simulink model "manipulator2"  (Simulink 8.8)
settings: Solver=FixedStepAuto  StartTime=0.0  StopTime=10.2557  FixedStep=0.001  RelTol=1e-3
settings Model: Creator=dell  LastModifiedBy=dell
settings DataIOCC: LimitDataPoints=off  SaveFormat=Dataset  SignalLoggingSaveFormat=Dataset
settings OptimizationCC: LifeSpan=auto
settings DebuggingCC: UnderspecifiedInitializationDetection=Simplified  MergeDetectMultiDrivingBlocksExec=error  FcnCallInpInsideContextMsg=error  StateNameClashWarn=none  SFUnexpectedBacktrackingDiag=error  SFNoUnconditionalDefaultTransitionDiag=error  SFExecutionAtInitializationDiag=warning
settings HardwareCC: ProdBitPerPointer=64  ProdBitPerSizeT=64  ProdBitPerPtrDiffT=64  ProdLargestAtomicFloat=Float  ProdIntDivRoundTo=Zero  ProdEndianess=LittleEndian  ProdWordSize=64  ProdHWDeviceType=Intel->x86-64 (Windows64)
settings ModelReferenceCC: PropagateSignalLabelsOutOfModel=on
settings GRTTargetCC: TargetLangStandard=C99 (ISO)  GeneratePreprocessorConditionals=Use local settings  CombineOutputUpdateFcns=on  GRTInterface=off
settings ConfigComp: CovMetricSettings=dwe  CovHtmlReporting=off  CovSaveCumulativeToWorkspaceVar=off  CovSaveSingleToWorkspaceVar=off  CovExternalEMLEnable=on

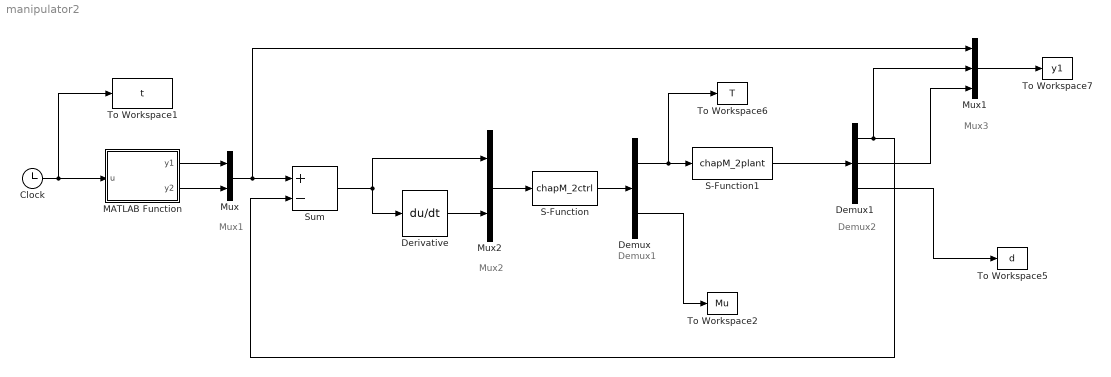
== system manipulator2 ==
  note: Demux2
  note: Mux3
  note: Demux1
  note: Mux2
  note: Mux1
  Clock : Clock
  Demux : Demux  Outputs=2
  Demux1 : Demux  Outputs=3
  Derivative : Derivative
  MATLAB Function : MATLAB Function  TreatAsAtomicUnit=on
  Mux : Mux  Inputs=2
  Mux1 : Mux  Inputs=3
  Mux2 : Mux  Inputs=2
  S-Function : S-Function  FunctionName=chapM_2ctrl  SFunctionDeploymentMode=off  EnableBusSupport=off
  S-Function1 : S-Function  FunctionName=chapM_2plant  SFunctionDeploymentMode=off  EnableBusSupport=off
  Sum : Sum  Inputs=+-  SaturateOnIntegerOverflow=on  InputSameDT=on  OutDataTypeStr=Inherit: Same as first input
  To Workspace1 : ToWorkspace  VariableName=t  SampleTime=-1
  To Workspace2 : ToWorkspace  VariableName=Mu  SampleTime=-1
  To Workspace5 : ToWorkspace  VariableName=d  SampleTime=-1
  To Workspace6 : ToWorkspace  VariableName=T  SampleTime=-1
  To Workspace7 : ToWorkspace  VariableName=y1  SampleTime=-1
  wires:
  MATLAB Function/2(y2) -> Mux/2
  MATLAB Function/1(y1) -> Mux/1
  S-Function/1 -> Demux/1
  Demux/1 -> To Workspace6/1, S-Function1/1
  S-Function1/1 -> Demux1/1
  Clock/1 -> To Workspace1/1, MATLAB Function/1(u)
  Mux2/1 -> S-Function/1
  Derivative/1 -> Mux2/2
  Mux1/1 -> To Workspace7/1
  Mux/1 -> Mux1/1, Sum/1
  Sum/1 -> Mux2/1, Derivative/1
  Demux/2 -> To Workspace2/1
  Demux1/3 -> To Workspace5/1
  Demux1/1 -> Mux1/2, Sum/2
  Demux1/2 -> Mux1/3

== matlab function MATLAB Function ==
  data: u input double; y1 output double; y2 output double
function [y1,y2]=fcn(u)
y1=sin(u);
y2=cos(u);
